simulink model "BinObserver"  (Simulink 5.0)
settings: Solver=FixedStepDiscrete  StartTime=0.0  StopTime=10  FixedStep=0.04  RelTol=1e-3
settings Model: LastModifiedBy=cvilas

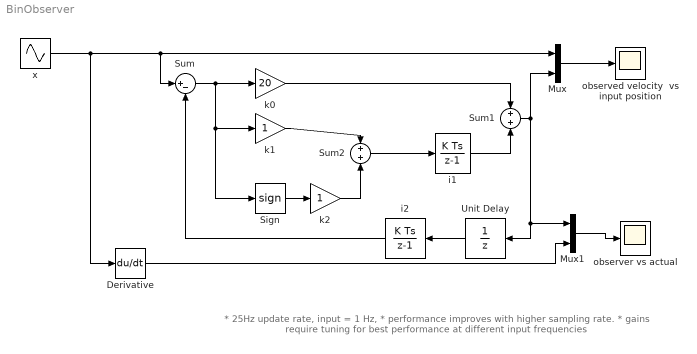
== system BinObserver ==
  note: * 25Hz update rate, input = 1 Hz,
      | * performance improves with higher sampling rate.
      | * gains require tuning for best performance at
      | different input frequencies
  Derivative : Derivative
  Mux : Mux  Inputs=2
  Mux1 : Mux  Inputs=2
  Sign : Signum
  Sum : Sum  Inputs=|+-  SaturateOnIntegerOverflow=on
  Sum1 : Sum  Inputs=+|+  SaturateOnIntegerOverflow=on
  Sum2 : Sum  Inputs=+|+  SaturateOnIntegerOverflow=on
  Unit Delay : UnitDelay  Orientation=left  SampleTime=-1
  i1 : DiscreteIntegrator  SampleTime=-1
  i2 : DiscreteIntegrator  Orientation=left  SampleTime=-1
  k0 : Gain  Gain=20  SaturateOnIntegerOverflow=on
  k1 : Gain  SaturateOnIntegerOverflow=on
  k2 : Gain  SaturateOnIntegerOverflow=on
  observed velocity  vs input position : Scope
      settings: YMin=-2.5  YMax=2.5  MaxDataPoints=100000
  observer vs actual : Scope
      settings: YMin=-15  YMax=15  MaxDataPoints=100000
  x : Sin  Amplitude=10  Frequency=2 * pi * 1.0  SampleTime=0.04
  wires:
  Sum/1 -> k0/1, k1/1, Sign/1
  k1/1 -> Sum2/1
  k2/1 -> Sum2/2
  Sign/1 -> k2/1
  Sum2/1 -> i1/1
  i1/1 -> Sum1/2
  k0/1 -> Sum1/1
  Sum1/1 -> Mux/2, Mux1/1, Unit Delay/1
  Mux/1 -> observed velocity  vs input position/1
  x/1 -> Mux/1, Sum/1, Derivative/1
  i2/1 -> Sum/2
  Mux1/1 -> observer vs actual/1
  Derivative/1 -> Mux1/2
  Unit Delay/1 -> i2/1
